simulink model "PID_saturated"  (R2025b)
settings: Solver=ode45  StartTime=0.0  StopTime=sim_stop_time  MaxStep=sim_step_time  RelTol=1e-8  AbsTol=1e-8
undefined symbols (not defined in the file): Bm, Jm, K, kd, ki, kp, LGain, Lm, ref_speed, Rm, sim_step_time, vref
libraries: slpidlib x1
settings Model: Creator=shashi  LastModifiedBy=shashi
settings SolverCC: AutoScaleAbsTol=off
settings DataIOCC: SaveOutput=off  SignalLogging=off  DSMLogging=off  SaveTime=off  ReturnWorkspaceOutputs=off

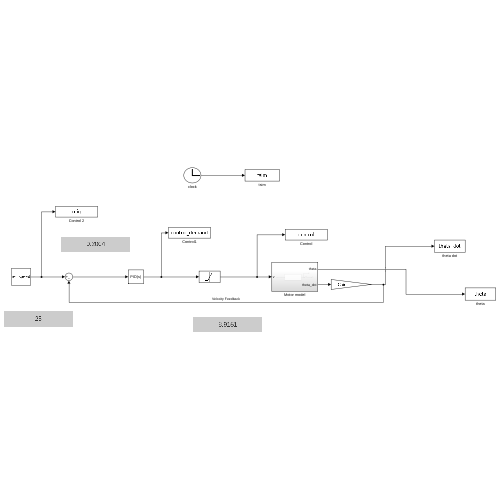
[thumbnail: Simulink's stored preview of the top-level diagram]
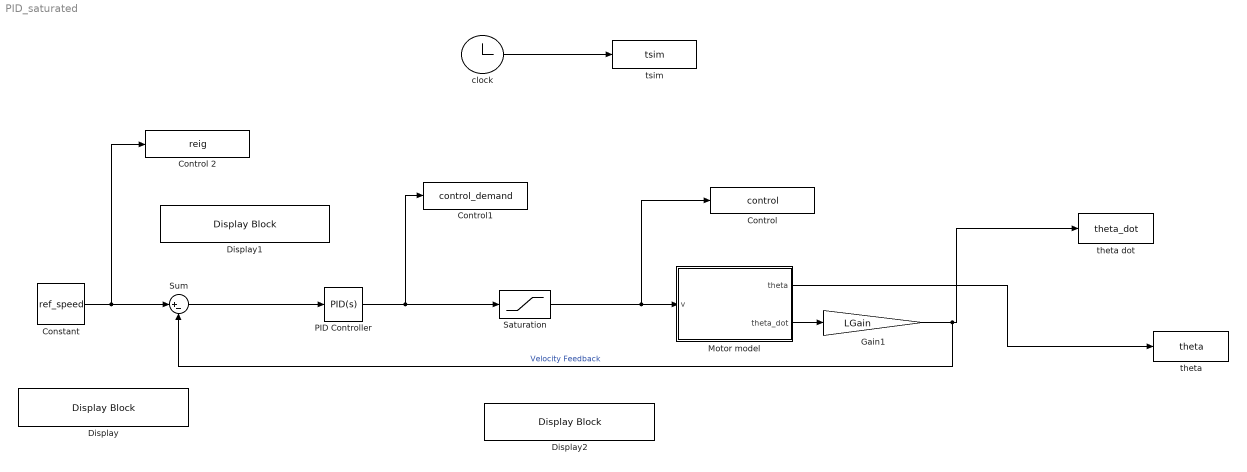
== system PID_saturated ==
  Constant : Constant  Value=ref_speed  SampleTime=sim_step_time
  Control : ToWorkspace  VariableName=control  SampleTime=sim_step_time
      settings: Save2DSignal=2-D array (concatenate along first dimension)
  Control 2 : ToWorkspace  VariableName=reig  SampleTime=sim_step_time
      settings: Save2DSignal=2-D array (concatenate along first dimension)
  Control1 : ToWorkspace  VariableName=control_demand  SampleTime=sim_step_time
      settings: Save2DSignal=2-D array (concatenate along first dimension)
  Display : DisplayBlock  LabelPosition=Hide  Transparency=1  GridColor=[0.502, 0.502, 0.502]
  Display1 : DisplayBlock  LabelPosition=Hide  Transparency=1  GridColor=[0.502, 0.502, 0.502]
  Display2 : DisplayBlock  LabelPosition=Hide  Transparency=1  GridColor=[0.502, 0.502, 0.502]
  Gain1 : Gain  Gain=LGain
  Motor model : Subsystem
  PID Controller : slpidlib/PID Controller  Controller=PID  Form=Parallel  TimeDomain=Continuous-time  UseExternalTs=off  SampleTime=-1  IntegratorMethod=Forward Euler  FilterMethod=Forward Euler  ControllerParametersSource=internal  P=kp  I=ki  UseKiTs=off  D=kd  UseExternalDerivativeSource=off  N=100  UseFilter=on  TunerSelectOption=Transfer Function Based (PID Tuner App)  InitialConditionSource=internal  InitialConditionForIntegrator=0  InitialConditionForFilter=0  DifferentiatorICPrevScaledInput=0  ExternalReset=none  TrackingMode=off  Kt=1  LimitOutput=off  SatLimitsSource=internal  UpperSaturationLimit=inf  LowerSaturationLimit=-inf  LinearizeAsGain=on  AntiWindupMode=none  Kb=1  LimitIntegrator=off  UpperIntegratorSaturationLimit=inf  LowerIntegratorSaturationLimit=-inf  POutMin=[]  POutMax=[]  IOutMin=[]  IOutMax=[]  DOutMin=[]  DOutMax=[]  NOutMin=[]  NOutMax=[]  SumOutMin=[]  SumOutMax=[]  SaturationOutMin=[]  SaturationOutMax=[]  PParamMin=[]  PParamMax=[]  IParamMin=[]  IParamMax=[]  DParamMin=[]  DParamMax=[]  NParamMin=[]  NParamMax=[]  KbParamMin=[]  KbParamMax=[]  KtParamMin=[]  KtParamMax=[]  KbOutMin=[]  KbOutMax=[]  KtOutMin=[]  KtOutMax=[]  IntegratorOutMin=[]  IntegratorOutMax=[]  FilterOutMin=[]  FilterOutMax=[]  SumI1OutMin=[]  SumI1OutMax=[]  SumI2OutMin=[]  SumI2OutMax=[]  SumI3OutMin=[]  SumI3OutMax=[]  SumI4OutMin=[]  SumI4OutMax=[]  SumDOutMin=[]  SumDOutMax=[]  DifferentiatorOutMin=[]  DifferentiatorOutMax=[]  FilterDiffOutCoefMin=[]  FilterDiffOutCoefMax=[]  ReciprocalOutMin=[]  ReciprocalOutMax=[]  SumDenOutMin=[]  SumDenOutMax=[]  SumNumOutMin=[]  SumNumOutMax=[]  DivideOutMin=[]  DivideOutMax=[]  UdiffTsProdOutMin=[]  UdiffTsProdOutMax=[]  NTsProdOutMin=[]  NTsProdOutMax=[]  UintegralTsProdOutMin=[]  UintegralTsProdOutMax=[]  UngainTsProdOutMin=[]  UngainTsProdOutMax=[]  ClampingZeroOutDataTypeStr=Inherit: Inherit via back propagation  ClampingZeroOutMin=[]  ClampingZeroOutMax=[]  FilterDenConstantOutDataTypeStr=Inherit: Inherit via back propagation  FilterDenConstantOutMin=[]  FilterDenConstantOutMax=[]  PCopyOutDataTypeStr=Inherit: Inherit via back propagation  PCopyOutMin=[]  PCopyOutMax=[]  NCopyOutDataTypeStr=Inherit: Inherit via back propagation  NCopyOutMin=[]  NCopyOutMax=[]  IntegratorContinuousStateAttributes=''  IntegratorStateMustResolveToSignalObject=off  IntegratorRTWStateStorageClass=Auto  FilterContinuousStateAttributes=''  FilterStateMustResolveToSignalObject=off  FilterRTWStateStorageClass=Auto  ParallelPVariant=InternalParameters  IdealPVariant=Disabled  IVariant=InternalParameters  DVariant=InternalParameters  IntegratorVariant=Continuous  SatVariant=Disabled  AWVariant=Passthrough  PCopyVariant=Disabled  TRVariant=Disabled  FdbkBlocksVariant=Forward  IdealPFdbkVariant=Disabled  SatFdbkVariant=Disabled  DerivativeFilterVariant=ContFilter  NVariant=InternalParameters  NCopyVariant=Disabled  FilterICVariant=InternalICsFilter  IntegratorICVariant=InternalICs  ExternalResetVariant=Disabled  TRSumVariant=Passthrough  SumFdbkVariant=Disabled  SumVariant=Sum_PID  TsampFilterVariant=InternalTs  TsampNgainVariant=Passthrough  TsampIntegralVariant=Disabled_SignalSpec  ExternalSaturationOutDataTypeStr=Inherit: Same as second input  DerivativeSourceVariant=ErrorSignal  PreIntVariant=InternalPreInt
  Saturation : Saturate  UpperLimit=+vref  LowerLimit=-vref
  Sum : Sum  Inputs=|+-
  clock : Clock
  theta : ToWorkspace  VariableName=theta  SampleTime=sim_step_time
      settings: Save2DSignal=2-D array (concatenate along first dimension)
  theta dot : ToWorkspace  VariableName=theta_dot  SampleTime=sim_step_time
      settings: Save2DSignal=2-D array (concatenate along first dimension)
  tsim : ToWorkspace  VariableName=tsim  SampleTime=sim_step_time
      settings: Save2DSignal=2-D array (concatenate along first dimension)
  wires:
  clock/1 -> tsim/1
  PID Controller/1 -> Control1/1, Saturation/1
  Motor model/2(theta_dot) -> Gain1/1
  Constant/1 -> Sum/1, Control 2/1
  Motor model/1(theta) -> theta/1
  Saturation/1 -> Motor model/1(v), Control/1
  Sum/1 -> PID Controller/1
  Gain1/1 -> theta dot/1, Sum/2  "Velocity Feedback"

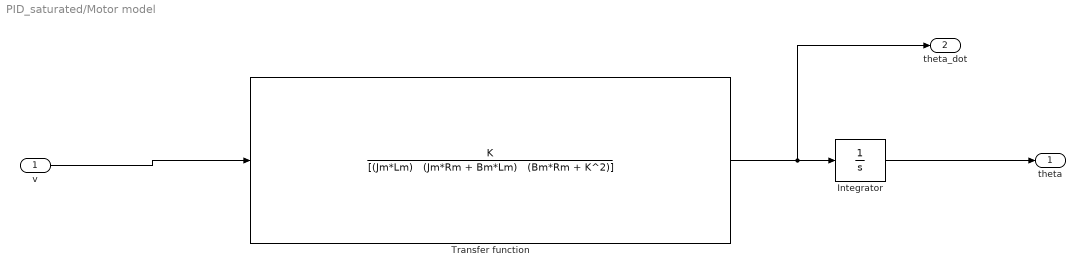
== system PID_saturated/Motor model ==
  v : Inport
  Integrator : Integrator
  Transfer function : TransferFcn  Numerator=K  Denominator="[(Jm*Lm)   (Jm*Rm + Bm*Lm)   (Bm*Rm + K^2)]"
  theta : Outport
  theta_dot : Outport  Port=2
  wires:
  v/1 -> Transfer function/1
  Transfer function/1 -> theta_dot/1, Integrator/1
  Integrator/1 -> theta/1
